simulink model "SimTrackFollowing5"  (Simulink 3.00)
settings: Solver=ode45  StartTime=0.0  StopTime=NmaxTs*Ts  RelTol=1e-3
values from neighbouring files (symbols this model uses):
  g_flutter = 1    [followdemo.m]
  g_rro = 1    [followdemo.m]
  g_sensor = 1    [followdemo.m]
  g_torque = 1    [followdemo.m]
  loopgain = 1+loopgain_pt(jj)    [evperf.m]
  Tc = Ts/2    [followdemo.m]
  Ts = PlantData.Ts    [followdemo.m]
undefined symbols (not defined in the file or in its folder): FlutterDist, ForceDist, RRO, SensorNoise
libraries: cstblocks x3
settings Model: LastModifiedBy=takeyori

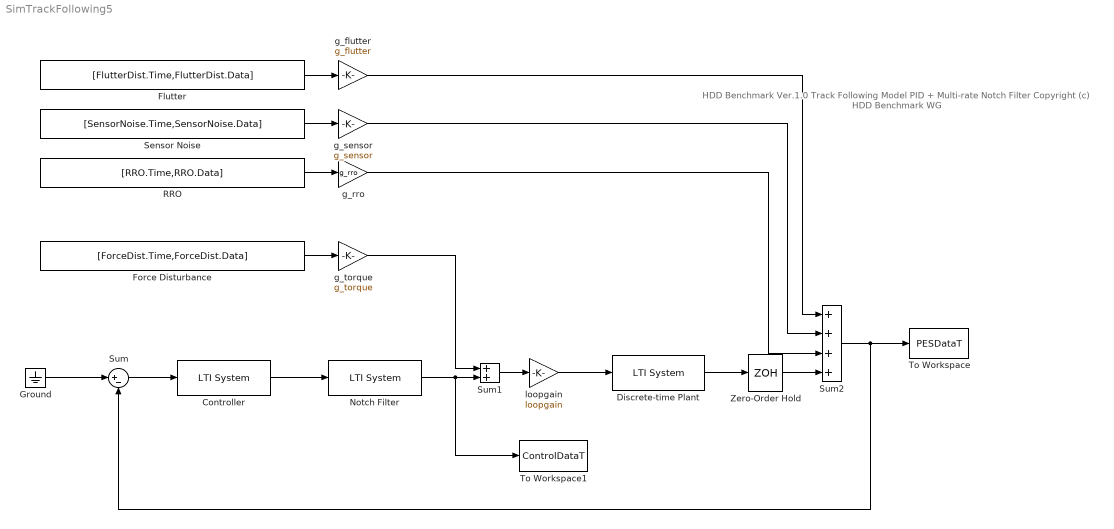
== system SimTrackFollowing5 ==
  note: HDD Benchmark Ver.1.0
      | Track Following Model
      | PID + Multi-rate Notch Filter
      | Copyright (c) HDD Benchmark WG
  Controller : cstblocks/LTI System  sys=sys_C1  IC=[0]
  Discrete-time Plant : cstblocks/LTI System  sys=sysd_P  IC=[0]
  Flutter : FromWorkspace  VariableName=[FlutterDist.Time,FlutterDist.Data]  SampleTime=FlutterDist.Ts  HoldFinalValue=off
  Force Disturbance : FromWorkspace  VariableName=[ForceDist.Time,ForceDist.Data]  SampleTime=ForceDist.Ts  HoldFinalValue=off
  Ground : Ground
  Notch Filter : cstblocks/LTI System  sys=sys_C2  IC=[0]
  RRO : FromWorkspace  VariableName=[RRO.Time,RRO.Data]  SampleTime=RRO.Ts  HoldFinalValue=off
  Sensor Noise : FromWorkspace  VariableName=[SensorNoise.Time,SensorNoise.Data]  SampleTime=SensorNoise.Ts  HoldFinalValue=off
  Sum : Sum  Inputs=|+-  SaturateOnIntegerOverflow=on
  Sum1 : Sum  Inputs=++  SaturateOnIntegerOverflow=on
  Sum2 : Sum  Inputs=+++|+  SaturateOnIntegerOverflow=on
  To Workspace : ToWorkspace  VariableName=PESDataT  SampleTime=Ts  SaveFormat=StructureWithTime
      settings: Buffer=NmaxTs
  To Workspace1 : ToWorkspace  VariableName=ControlDataT  SampleTime=Tc  SaveFormat=StructureWithTime
      settings: Buffer=NmaxTc
  Zero-Order Hold : ZeroOrderHold  SampleTime=Ts
  g_flutter : Gain  Gain=g_flutter  SaturateOnIntegerOverflow=on
  g_rro : Gain  Gain=g_rro  SaturateOnIntegerOverflow=on
  g_sensor : Gain  Gain=g_sensor  SaturateOnIntegerOverflow=on
  g_torque : Gain  Gain=g_torque  SaturateOnIntegerOverflow=on
  loopgain : Gain  Gain=loopgain  SaturateOnIntegerOverflow=on
  wires:
  Flutter/1 -> g_flutter/1
  Sensor Noise/1 -> g_sensor/1
  RRO/1 -> g_rro/1
  Controller/1 -> Notch Filter/1
  Sum1/1 -> loopgain/1
  Sum/1 -> Controller/1
  loopgain/1 -> Discrete-time Plant/1
  Force Disturbance/1 -> g_torque/1
  g_torque/1 -> Sum1/1
  Ground/1 -> Sum/1
  Discrete-time Plant/1 -> Zero-Order Hold/1
  Zero-Order Hold/1 -> Sum2/4
  Sum2/1 -> To Workspace/1, Sum/2
  Notch Filter/1 -> Sum1/2, To Workspace1/1
  g_rro/1 -> Sum2/3
  g_sensor/1 -> Sum2/2
  g_flutter/1 -> Sum2/1
